simulink model "ddcm"  (R2019b)
settings: Solver=FixedStepAuto  StartTime=0.0  StopTime=10.0  FixedStep=0.1  RelTol=1e-3
settings Model: Creator=ADEMATO1  LastModifiedBy=EMORAI12
settings SolverCC: PositivePriorityOrder=on  AutoInsertRateTranBlk=on  InsertRTBMode=Always

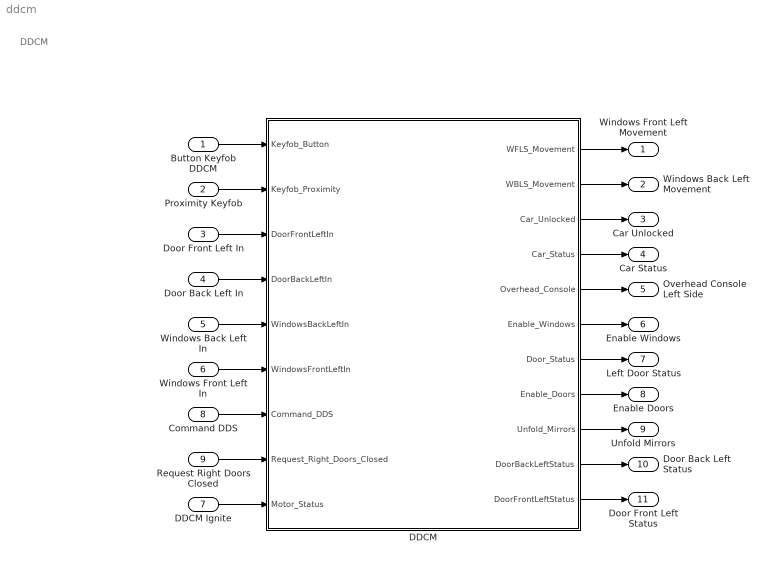
== system ddcm ==
  note: DDCM
  Button Keyfob DDCM : Inport
  Proximity Keyfob : Inport  Port=2
  Door Front Left In : Inport  Port=3
  Door Back Left In : Inport  Port=4
  Windows Back Left In : Inport  Port=5
  Windows Front Left In : Inport  Port=6
  DDCM Ignite : Inport  Port=7
  Command DDS : Inport  Port=8
  Request Right Doors Closed : Inport  Port=9
  DDCM : Stateflow chart  TreatAsAtomicUnit=on
  Windows Front Left Movement : Outport
  Windows Back Left Movement : Outport  Port=2
  Car Unlocked : Outport  Port=3
  Car Status : Outport  Port=4
  Overhead Console Left Side : Outport  Port=5
  Enable Windows : Outport  Port=6
  Left Door Status : Outport  Port=7
  Enable Doors : Outport  Port=8
  Unfold Mirrors : Outport  Port=9
  Door Back Left Status : Outport  Port=10
  Door Front Left Status : Outport  Port=11
  wires:
  DDCM Ignite/1 -> DDCM/9(Motor_Status)
  DDCM/8(Enable_Doors) -> Enable Doors/1
  DDCM/7(Door_Status) -> Left Door Status/1
  Windows Back Left In/1 -> DDCM/5(WindowsBackLeftIn)
  Door Back Left In/1 -> DDCM/4(DoorBackLeftIn)
  DDCM/6(Enable_Windows) -> Enable Windows/1
  DDCM/2(WBLS_Movement) -> Windows Back Left Movement/1
  DDCM/1(WFLS_Movement) -> Windows Front Left Movement/1
  Request Right Doors Closed/1 -> DDCM/8(Request_Right_Doors_Closed)
  DDCM/3(Car_Unlocked) -> Car Unlocked/1
  DDCM/5(Overhead_Console) -> Overhead Console Left Side/1
  Command DDS/1 -> DDCM/7(Command_DDS)
  DDCM/9(Unfold_Mirrors) -> Unfold Mirrors/1
  DDCM/4(Car_Status) -> Car Status/1
  Door Front Left In/1 -> DDCM/3(DoorFrontLeftIn)
  Proximity Keyfob/1 -> DDCM/2(Keyfob_Proximity)
  Button Keyfob DDCM/1 -> DDCM/1(Keyfob_Button)
  Windows Front Left In/1 -> DDCM/6(WindowsFrontLeftIn)
  DDCM/10(DoorBackLeftStatus) -> Door Back Left Status/1
  DDCM/11(DoorFrontLeftStatus) -> Door Front Left Status/1

== stateflow chart ddcm/DDCM ==
  state Left_Doors_Enable
    state Windows_Switch_When_TOff [parallel]
      during:
      if (aux2==1 &&  time ==1)
      WFLS_Movement = WindowsFrontLeftIn;
      WBLS_Movement = WindowsBackLeftIn;
      else
      WFLS_Movement = -1;
      WBLS_Movement = -1;
      end
      settings: executionOrder=2
    state Left_Doors_Enable_2 [parallel]
      entry:
      Car_Status = 0;
      during:
      if (Enable_Doors == 1)
      DFLS = DoorFrontLeftIn;
      DBLS = DoorBackLeftIn;
      end
      if (DFLS == 1 | DBLS == 1)
      Overhead_Console = 1;
      Door_Status = 1;
      else
      Door_Status = 0;
      Overhead_Console = 0;
      end
      if (DFLS == 1)
      DoorFrontLeftStatus = 1;
      else
      DoorFrontLeftStatus = 0;
      end
      if (DBLS == 1)
      DoorBackLeftStatus = 1;
      else
      DoorBackLeftStatus = 0;
      end
      settings: executionOrder=1
    state count [parallel]
      settings: executionOrder=3
      state state_count
        entry :
        time =0;
        during :
        if(aux2==1)
        time =1;
        else
        time =0;
        end
      state state_count1
        during :
      (default) -> state_count
      state_count -> state_count1 : [time==1]
      state_count1 -> state_count : [after(10,sec)]{ aux2=0}
  state State_Unlock_DDCM
    entry:
    Car_Unlocked = 1;
    Unfold_Mirrors = 1;
    Enable_Doors = 1;
  state Wait_Car_On
    entry:
    Car_Status = 1;
    aux2 = 0;
    during:
    if ((Enable_Windows == 1 ||  DDS < 7) && Enable_Doors == 1)
    AUX = 4 ;
    elseif  (Enable_Windows == 1 | DDS < 7)
    AUX = 1;
    elseif (Enable_Doors == 1)
    AUX = 3;
    end
  state Lock_Unlock
    entry:
    DFLS = 0;
    DBLS = 0;
    Door_Status = 0;
    WFLS_Movement = -1;
    WBLS_Movement = -1;
    Close_Windows = 1;
    aux2 = 0;
    Enable_Doors = 0;
  state Car_Ignite
    entry:
    Enable_Windows = 1;
    DDS = 0;
    Ignite = 1;
    exit :
    aux2 = 0;
  state Windows_Closed
    entry:
    WFLS_Movement = -1;
    WBLS_Movement = -1;
    Close_Windows = 0;
  state DDS_Enable
    entry :
    AUX  = 0 ;
    during:
    DDS = Command_DDS;
    if (DDS == 1)
    Enable_Windows = 1;
    elseif (DDS == 6)
    Enable_Windows = 0;
    WBLS_Movement = -1;
    WBLS_Movement = -1;
    elseif (DDS == 2)
    Unfold_Mirrors = 0;
    elseif (DDS == 3)
    Unfold_Mirrors = 1;
    elseif (DDS == 4)
    Enable_Doors = 0;
    elseif (DDS == 5)
    Enable_Doors = 1;
    end
    AUX = 2;
  state Windows_Update
  state Open_WFLS
    entry:
    WFLS_Movement = 0;
  state Open_WBLS
    entry:
    WBLS_Movement = 0;
  state Windows_Control
    entry:
    aux1 = 0;
    WFLS = WindowsFrontLeftIn;
    WBLS = WindowsBackLeftIn;
    during:
    aux1 = 1;
  state Left_Doors_Control
    entry:
    DFLS = DoorFrontLeftIn;
    DBLS = DoorBackLeftIn;
    during:
    if (DFLS == 1 | DBLS == 1)
    Overhead_Console = 1;
    Door_Status = 1;
    elseif (DFLS == 0 & DBLS == 0)
    Overhead_Console = 0;
    Door_Status = 0;
    end
    if (DFLS == 1)
    DoorFrontLeftStatus = 1;
    else
    DoorFrontLeftStatus = 0;
    end
    if (DBLS == 1)
    DoorBackLeftStatus = 1;
    else
    DoorBackLeftStatus = 0;
    end
    if (AUX ==3 | AUX == 5)
    AUX = 2;
    elseif (AUX==4)
    AUX=5;
    end
  state Close_WBLS
    entry:
    WBLS_Movement = 1;
  state Close_WFLS
    entry:
    WFLS_Movement = 1;
  state Closing_Windows
    entry:
    WFLS_Movement = 1;
    WBLS_Movement = 1;
  state State_Lock_DDCM
    entry:
    if (DFLS == 0 & DBLS == 0 & Request_Right_Doors_Closed == 1)
    Car_Unlocked = 0;
    Unfold_Mirrors = 0;
    Enable_Doors = 0;
    Close_Windows = 1;
    Enable_Doors = 0;
    else
    Enable_Doors = 1;
    Close_Windows = 0;
    Car_Unlocked = 1;
    end
  Wait_Car_On -> Left_Doors_Enable [order 1] : [Motor_Status == 0]{aux2=1}
  State_Unlock_DDCM -> Left_Doors_Enable : [Enable_Doors == 1]
  State_Lock_DDCM -> Left_Doors_Enable [order 2] : [Car_Unlocked == 1 & Close_Windows == 0]
  Left_Doors_Enable -> State_Lock_DDCM [order 2] : [Keyfob_Button == 1]
  Left_Doors_Enable -> Car_Ignite [order 1] : [Motor_Status == 1]
  (default) -> Lock_Unlock
  Lock_Unlock -> State_Unlock_DDCM [order 1] : [Keyfob_Button == 2]
  Wait_Car_On -> DDS_Enable [order 4] : after(200,msec)
  Windows_Closed -> State_Unlock_DDCM : [Keyfob_Button == 2]
  Lock_Unlock -> State_Lock_DDCM [order 2] : [Keyfob_Button == 1]
  Wait_Car_On -> Windows_Control [order 2] : [Enable_Windows == 1 & AUX == 1]
  Car_Ignite -> DDS_Enable : [Ignite == 1]
  DDS_Enable -> Wait_Car_On : [AUX==2]
  Wait_Car_On -> Left_Doors_Control [order 3] : [AUX == 3 || AUX == 4]
  (junction 396) -> Windows_Update [order 3] : [WBLS == -1] {WBLS_Movement = -1}
  (junction 412) -> (junction 396) [order 3] : [WFLS == -1] {WFLS_Movement = -1}
  Closing_Windows -> Windows_Closed : after(5,sec)
  Open_WBLS -> Windows_Update
  Open_WFLS -> (junction 396)
  (junction 396) -> Open_WBLS [order 1] : [WBLS == 0]
  Close_WFLS -> (junction 396)
  (junction 396) -> Close_WBLS [order 2] : [WBLS == 1]
  Windows_Control -> (junction 412) : [aux1 == 1]
  (junction 412) -> Open_WFLS [order 1] : [WFLS == 0]
  (junction 412) -> Close_WFLS [order 2] : [WFLS == 1]
  Left_Doors_Control -> Windows_Control [order 2] : [AUX==5 & Enable_Windows == 1]
  Close_WBLS -> Windows_Update
  Windows_Update -> DDS_Enable : after (200,msec)
  (junction 418) -> Closing_Windows : after(3,sec)
  State_Lock_DDCM -> (junction 418) [order 1] : [Close_Windows == 1]
  Left_Doors_Control -> DDS_Enable [order 1] : [AUX == 2 & Enable_Doors == 1]
  data: BRWSdot local; BRWS local; PWS local; PWSdot local; BLWS local; BLWSdot local; DWS local; Fold_Mirrors_Key local; DDS_Command local; DDS local; Keyfob_Button input; Keyfob_Proximity input; DoorFrontLeftIn input; DoorBackLeftIn input; WindowsBackLeftIn input; WindowsFrontLeftIn input; Command_DDS input; Request_Right_Doors_Closed input; WFLS_Movement output; WBLS_Movement output; Car_Unlocked output; Car_Status output; Overhead_Console output; WFLS local; WBLS local; Ignite local; DFLS local; DBLS local; Enable_Windows output; Close_Windows local; Door_Status output; aux2 local; aux1 local; AUX local; Enable_Doors output; Unfold_Mirrors output; Motor_Status input; time local; DoorBackLeftStatus output; DoorFrontLeftStatus output
